simulink model "B_Model"  (R2023b)
settings: Solver=ode45  StartTime=0.0  StopTime=time  MaxStep=0.001  RelTol=1e-3  EnableMultiTasking=on
values from neighbouring files (symbols this model uses):
  A = [0 1 0 ... (first row only)    [tf2ss_3rzad.m]
  h = h'    [lab5.m]
  t1 = 2    [lab5.m]
  xo = 1    [lab5.m]
  xo_obs = 0    [lab5.m]
undefined symbols (not defined in the file or in its folder): B, C
settings Model: Creator=Rafal  LastModifiedBy=pc
settings SolverCC: AlgebraicLoopSolver=TrustRegion
settings DataIOCC: SaveFormat=Array  ReturnWorkspaceOutputs=off
settings OptimizationCC: LifeSpan=inf
settings DebuggingCC: SolverPrmCheckMsg=warning  UnconnectedInputMsg=warning  UnconnectedOutputMsg=warning  UnconnectedLineMsg=warning  SFUnexpectedBacktrackingDiag=warning  SFNoUnconditionalDefaultTransitionDiag=warning  SFExecutionAtInitializationDiag=none  ArithmeticOperatorsInVariantConditions=warning
settings HardwareCC: ProdBitPerPointer=32  ProdBitPerSizeT=32  ProdBitPerPtrDiffT=32  ProdLargestAtomicFloat=None  ProdIntDivRoundTo=Undefined  ProdEndianess=Unspecified  ProdWordSize=32  ProdHWDeviceType=32-bit Generic
settings ModelReferenceCC: PropagateSignalLabelsOutOfModel=off
settings SFSimCC: SimUseLocalCustomCode=off  CustomCodeUndefinedFunction=UseInterfaceOnly
settings RTWCC: RTWUseLocalCustomCode=off
settings CodeAppCC: StateflowObjectComments=on
settings GRTTargetCC: TargetLangStandard=C89/C90 (ANSI)
settings ConfigComp: CovMetricSettings=dw  CovSaveCumulativeToWorkspaceVar=on  CovSaveSingleToWorkspaceVar=on  CovExternalEMLEnable=off  CovSFcnEnable=off

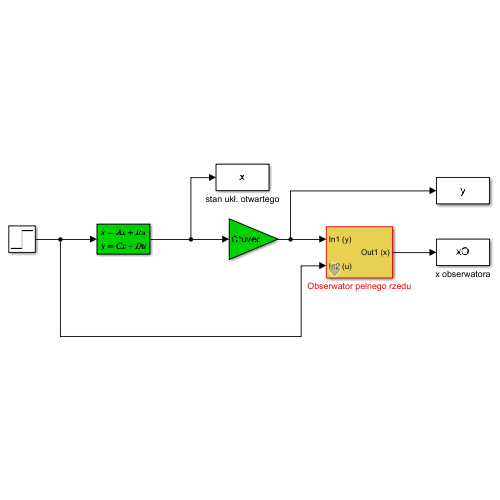
[thumbnail: Simulink's stored preview of the top-level diagram]
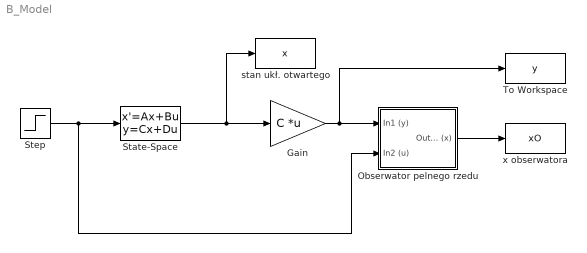
== system B_Model ==
  Gain : Gain  Gain=C  Multiplication=Matrix(K*u) (u vector)  SaturateOnIntegerOverflow=on  OutDataTypeStr=Inherit: Same as input  ParamDataTypeStr=Inherit: Same as input
  Obserwator pelnego rzedu : Subsystem  mask{H=h, xo_obs=xo_obs}
      mask prompts: xo_obs "war. poczakowy x(0)"
  State-Space : StateSpace  A=A  B=B  C=eye(3)  D=zeros(3,1)  InitialCondition=xo
  Step : Step  Time=t1  After=u  SampleTime=0
  To Workspace : ToWorkspace  VariableName=y  SampleTime=-1
  stan ukł. otwartego : ToWorkspace  VariableName=x  SampleTime=-1
  x obserwatora : ToWorkspace  VariableName=xO  SampleTime=-1
  wires:
  State-Space/1 -> Gain/1, stan ukł. otwartego/1
  Gain/1 -> To Workspace/1, Obserwator pelnego rzedu/1(In1 (y))
  Obserwator pelnego rzedu/1(Out1 (x)) -> x obserwatora/1
  Step/1 -> State-Space/1, Obserwator pelnego rzedu/2(In2 (u))

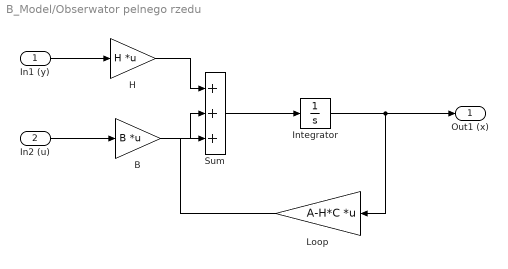
== system B_Model/Obserwator pelnego rzedu ==
  In1 (y) : Inport
  In2 (u) : Inport  Port=2
  B : Gain  Gain=B  Multiplication=Matrix(K*u) (u vector)  SaturateOnIntegerOverflow=on  OutDataTypeStr=Inherit: Same as input  ParamDataTypeStr=Inherit: Same as input
  H : Gain  Gain=H  Multiplication=Matrix(K*u) (u vector)  SaturateOnIntegerOverflow=on  OutDataTypeStr=Inherit: Same as input  ParamDataTypeStr=Inherit: Same as input
  Integrator : Integrator  InitialCondition=xo_obs
  Loop : Gain  Gain=A-H*C  Multiplication=Matrix(K*u) (u vector)  SaturateOnIntegerOverflow=on  OutDataTypeStr=Inherit: Same as input  ParamDataTypeStr=Inherit: Same as input
  Sum : Sum  Inputs=|+++  SaturateOnIntegerOverflow=on
  Out1 (x) : Outport
  wires:
  Sum/1 -> Integrator/1
  Integrator/1 -> Loop/1, Out1 (x)/1
  Loop/1 -> Sum/3
  B/1 -> Sum/2
  H/1 -> Sum/1
  In1 (y)/1 -> H/1
  In2 (u)/1 -> B/1
